simulink model "ProblemSet2"  (R2022a)
settings: Solver=VariableStepAuto  StartTime=0.0  StopTime=10.0  RelTol=1e-3
undefined symbols (not defined in the file): gray
libraries: simulink x4, matrix_library x2, dspindex x2, visiontextngfix x1, visionsources x1
settings Model: Creator=DT  LastModifiedBy=DT

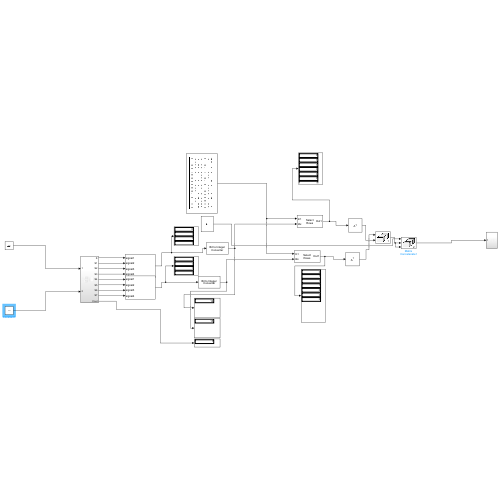
[thumbnail: Simulink's stored preview of the top-level diagram]
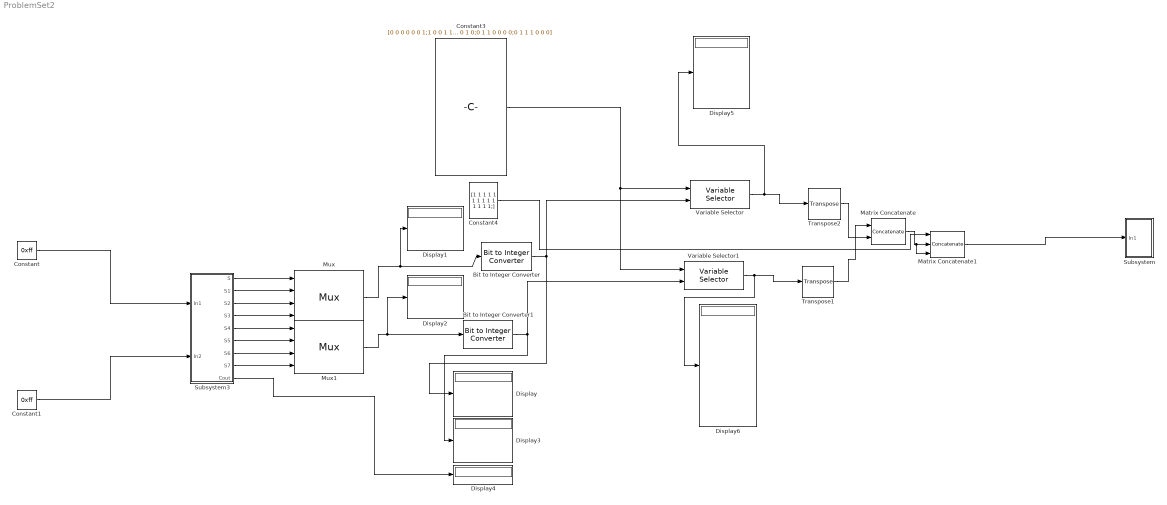
== system ProblemSet2 ==
  Bit to Integer Converter : simulink/Logic and Bit Operations/Bit to Integer Converter  nbits=4  bitOrder=LSB first  signedOutputValues=Unsigned  outDtype=Inherit via internal rule  outDtypeSigned=Inherit via internal rule
      settings: SourceProductBaseCode=SL
  Bit to Integer Converter1 : simulink/Logic and Bit Operations/Bit to Integer Converter  nbits=4  bitOrder=LSB first  signedOutputValues=Unsigned  outDtype=Inherit via internal rule  outDtypeSigned=Inherit via internal rule
      settings: SourceProductBaseCode=SL
  Constant : Constant  Value=0xff
  Constant1 : Constant  Value=0xff
  Constant3 : Constant  Value=[0 0 0 0 0 0 1;1 0 0 1 1 1 1;0 0 1 0 0 1 0;0 0 0 0 1 1 0;1 0 0 1 1 0 0;0 1 0 0 1 0 0 ;0 1 0 0 0 0 0;0 0 0 1 1 1 1;0 0 0 0 0 0 0;0 0 0 0 1 0 0;0 0 0 1 0 0 0;1 1 0 0 0 0 0;0 1 1 0 0 0 1;1 0 0 0 0 1 0;0 1 1 0 0 0 0;0 1 1 1 0 0 0]
  Constant4 : Constant  Value=[1 1 1 1 1 1 1 1 1 1 1 1 1 1;]
  Display{,1..6} (7 alike) : Display
      Display settings: Decimation=8
      Display3 settings: Decimation=8
  Matrix Concatenate : Concatenate  Mode=Multidimensional array
  Matrix Concatenate1 : Concatenate  NumInputs=3  Mode=Multidimensional array  ConcatenateDimension=2
  Mux : Mux
      settings: DisplayOption=signals
  Mux1 : Mux
      settings: DisplayOption=signals
  Subsystem : Subsystem
  Subsystem3 : Subsystem
  Transpose1 : matrix_library/Transpose
      settings: SourceProductBaseCode=SL
  Transpose2 : matrix_library/Transpose
      settings: SourceProductBaseCode=SL
  Variable Selector : dspindex/Variable Selector  NumInputs=1  rowsOrCols=Rows  IdxMode=Variable  Elements=[1 3]  ZerOneIdxMode=Zero-based  errmode=Clip Index  FillMode=on  FillValues=0
  Variable Selector1 : dspindex/Variable Selector  NumInputs=1  rowsOrCols=Rows  IdxMode=Variable  Elements=[1 3]  ZerOneIdxMode=Zero-based  errmode=Clip Index  FillMode=on  FillValues=0
  wires:
  Constant/1 -> Subsystem3/1(In1)
  Constant1/1 -> Subsystem3/2(In2)
  Subsystem3/1(S) -> Mux/1
  Subsystem3/2(S1) -> Mux/2
  Subsystem3/3(S2) -> Mux/3
  Subsystem3/4(S3) -> Mux/4
  Subsystem3/8(S7) -> Mux1/4
  Subsystem3/5(S4) -> Mux1/1
  Subsystem3/6(S5) -> Mux1/2
  Subsystem3/7(S6) -> Mux1/3
  Mux1/1 -> Display2/1, Bit to Integer Converter1/1
  Bit to Integer Converter/1 -> Display/1, Variable Selector/2
  Mux/1 -> Display1/1, Bit to Integer Converter/1
  Bit to Integer Converter1/1 -> Display3/1, Variable Selector1/2
  Subsystem3/9(Cout) -> Display4/1
  Constant3/1 -> Variable Selector1/1, Variable Selector/1
  Variable Selector/1 -> Display5/1, Transpose2/1
  Variable Selector1/1 -> Display6/1, Transpose1/1
  Transpose2/1 -> Matrix Concatenate/2
  Transpose1/1 -> Matrix Concatenate/1
  Matrix Concatenate/1 -> Matrix Concatenate1/3, Matrix Concatenate1/2
  Constant4/1 -> Matrix Concatenate1/1
  Matrix Concatenate1/1 -> Subsystem/1(In1)

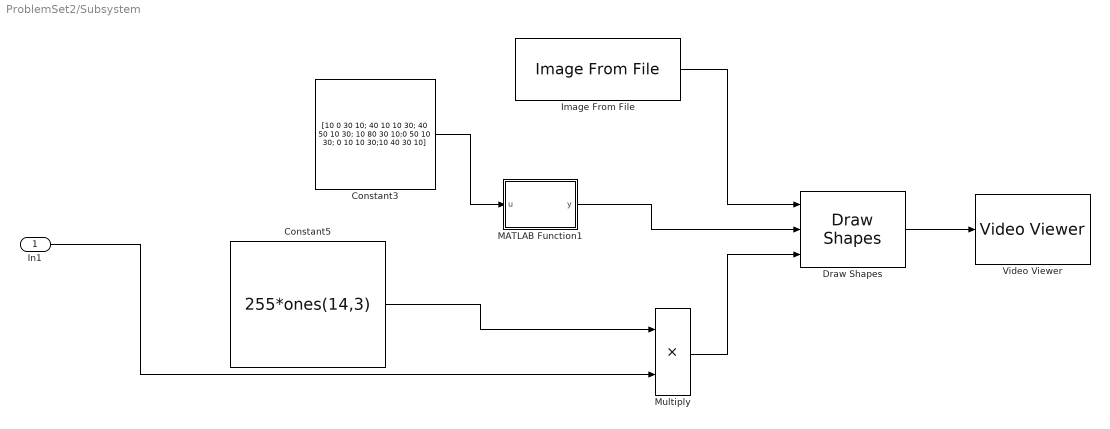
== system ProblemSet2/Subsystem ==
  In1 : Inport
  Constant3 : Constant  Value="[10 0  30 10; 40 10 10 30; 40 50 10 30; 10 80 30 10;0 50 10 30; 0 10 10 30;10 40 30 10]"  VectorParams1D=off
  Constant5 : Constant  Value=255*ones(14,3)
  Draw Shapes : visiontextngfix/Draw Shapes  shape=Rectangles  fill=on  lineWidth=1  fillClrSource=Input port  display=Black  intensity=200  color=[200 255 100]  opacity=0.6  viewport=Entire image  antialiasing=off  inType=Obsolete  imagePorts=One multidimensional signal  roundingMode=Floor  overflowMode=off  memoryMode=Specify word length  memoryWordLength=16  prodOutputMode=Binary point scaling  prodOutputWordLength=32  prodOutputFracLength=14  memoryFracLength=14
  Image From File : visionsources/Image From File  Tag=vipblks_nd  FileName=C:\Users\DT\Downloads\WhiteBackground.png  Ts=inf  imagePorts=One multidimensional signal  OutPortLabels=R|G|B  ImageDataType=double  sdImageDataType=uint(8)  Signed=on  WordLength=16  FractionLengthMode=User-defined  FractionLength=15
  MATLAB Function1 : MATLAB Function  TreatAsAtomicUnit=on
  Multiply : Product
  Video Viewer : VideoViewer  colormapValue=gray(256)  FigPos=[1 814 1536 716]
  wires:
  Constant5/1 -> Multiply/1
  Draw Shapes/1 -> Video Viewer/1
  MATLAB Function1/1(y) -> Draw Shapes/2
  In1/1 -> Multiply/2
  Image From File/1 -> Draw Shapes/1
  Constant3/1 -> MATLAB Function1/1(u)
  Multiply/1 -> Draw Shapes/3

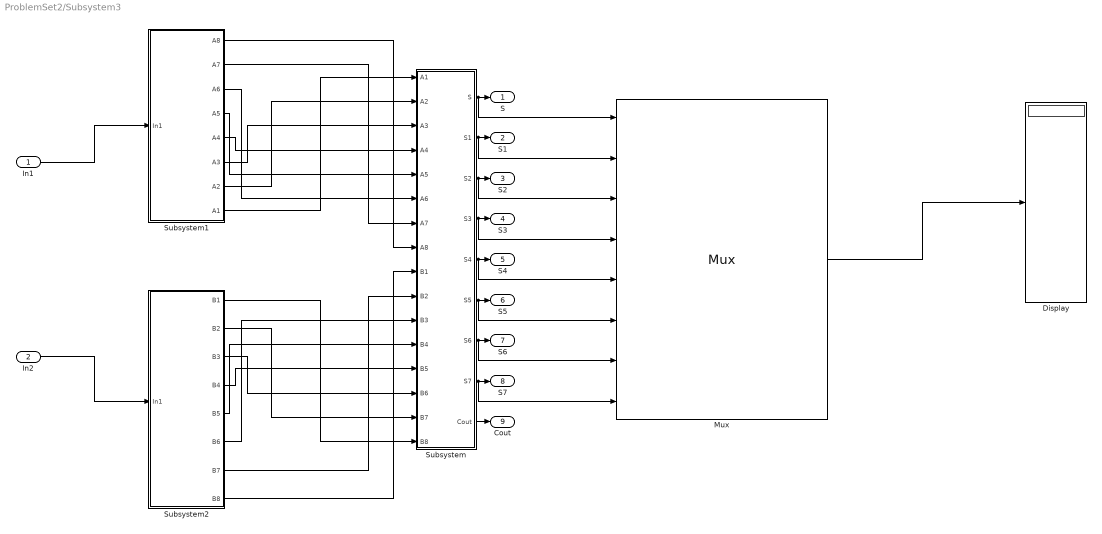
== system ProblemSet2/Subsystem3 ==
  In1 : Inport
  In2 : Inport  Port=2
  Display : Display
  Mux : Mux  Inputs=8
  Subsystem : Subsystem
  Subsystem1 : Subsystem
  Subsystem2 : Subsystem
  S : Outport
  S1 : Outport  Port=2
  S2 : Outport  Port=3
  S3 : Outport  Port=4
  S4 : Outport  Port=5
  S5 : Outport  Port=6
  S6 : Outport  Port=7
  S7 : Outport  Port=8
  Cout : Outport  Port=9
  wires:
  Subsystem/6(S5) -> Mux/6, S5/1
  Subsystem/4(S3) -> Mux/4, S3/1
  In1/1 -> Subsystem1/1(In1)
  In2/1 -> Subsystem2/1(In1)
  Subsystem/5(S4) -> Mux/5, S4/1
  Subsystem/7(S6) -> Mux/7, S6/1
  Subsystem/9(Cout) -> Cout/1
  Subsystem/8(S7) -> Mux/8, S7/1
  Subsystem/2(S1) -> Mux/2, S1/1
  Subsystem/3(S2) -> Mux/3, S2/1
  Subsystem/1(S) -> Mux/1, S/1
  Mux/1 -> Display/1
  Subsystem1/8(A1) -> Subsystem/1(A1)
  Subsystem1/7(A2) -> Subsystem/2(A2)
  Subsystem1/6(A3) -> Subsystem/3(A3)
  Subsystem1/5(A4) -> Subsystem/4(A4)
  Subsystem1/4(A5) -> Subsystem/5(A5)
  Subsystem1/3(A6) -> Subsystem/6(A6)
  Subsystem1/2(A7) -> Subsystem/7(A7)
  Subsystem1/1(A8) -> Subsystem/8(A8)
  Subsystem2/1(B1) -> Subsystem/16(B8)
  Subsystem2/2(B2) -> Subsystem/15(B7)
  Subsystem2/3(B3) -> Subsystem/14(B6)
  Subsystem2/4(B4) -> Subsystem/13(B5)
  Subsystem2/5(B5) -> Subsystem/12(B4)
  Subsystem2/6(B6) -> Subsystem/11(B3)
  Subsystem2/7(B7) -> Subsystem/10(B2)
  Subsystem2/8(B8) -> Subsystem/9(B1)

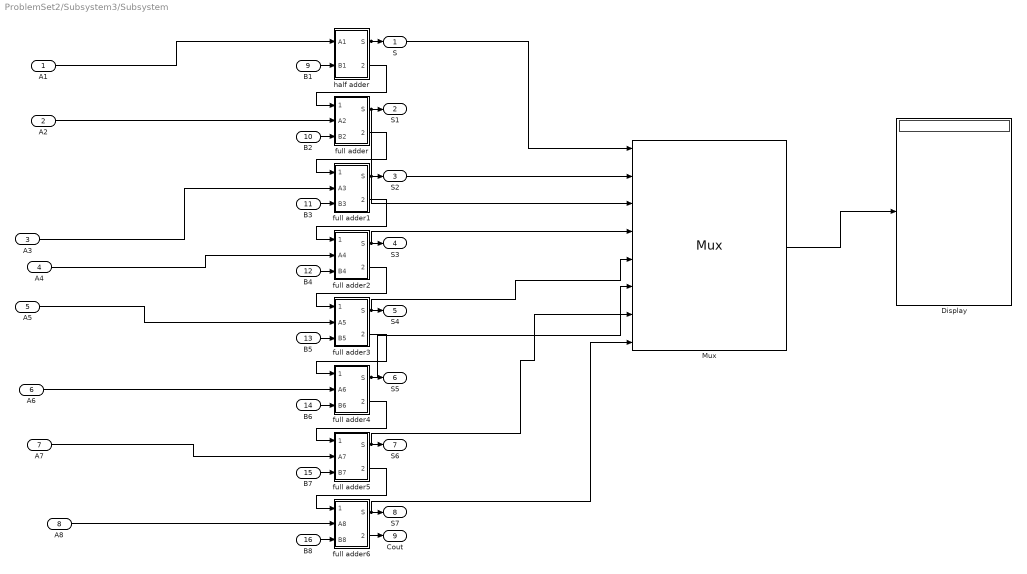
== system ProblemSet2/Subsystem3/Subsystem ==
  A1 : Inport
  A2 : Inport  Port=2
  A3 : Inport  Port=3
  A4 : Inport  Port=4
  A5 : Inport  Port=5
  A6 : Inport  Port=6
  A7 : Inport  Port=7
  A8 : Inport  Port=8
  B1 : Inport  Port=9
  B2 : Inport  Port=10
  B3 : Inport  Port=11
  B4 : Inport  Port=12
  B5 : Inport  Port=13
  B6 : Inport  Port=14
  B7 : Inport  Port=15
  B8 : Inport  Port=16
  Display : Display
  Mux : Mux  Inputs=8
  full adder : Subsystem
  full adder1 : Subsystem
  full adder2 : Subsystem
  full adder3 : Subsystem
  full adder4 : Subsystem
  full adder5 : Subsystem
  full adder6 : Subsystem
  half adder : Subsystem
  S : Outport
  S1 : Outport  Port=2
  S2 : Outport  Port=3
  S3 : Outport  Port=4
  S4 : Outport  Port=5
  S5 : Outport  Port=6
  S6 : Outport  Port=7
  S7 : Outport  Port=8
  Cout : Outport  Port=9
  wires:
  A7/1 -> full adder5/2(A7)
  A8/1 -> full adder6/2(A8)
  full adder6/1(S) -> Mux/8, S7/1
  full adder1/2(Cout) -> full adder2/1(Cin)
  full adder4/2(Cout) -> full adder5/1(Cin)
  half adder/2(Cout) -> full adder/1(Cin)
  A6/1 -> full adder4/2(A6)
  full adder2/2(Cout) -> full adder3/1(Cin)
  full adder5/2(Cout) -> full adder6/1(Cin)
  full adder/2(Cout) -> full adder1/1(Cin)
  full adder2/1(S) -> Mux/4, S3/1
  A3/1 -> full adder1/2(A3)
  full adder3/2(Cout) -> full adder4/1(Cin)
  A2/1 -> full adder/2(A2)
  A1/1 -> half adder/1(A1)
  A4/1 -> full adder2/2(A4)
  full adder/1(S) -> Mux/2, S1/1
  B3/1 -> full adder1/3(B3)
  A5/1 -> full adder3/2(A5)
  B6/1 -> full adder4/3(B6)
  full adder4/1(S) -> Mux/6, S5/1
  B7/1 -> full adder5/3(B7)
  half adder/1(S) -> Mux/1, S/1
  full adder5/1(S) -> Mux/7, S6/1
  full adder6/2(Cout) -> Cout/1
  B1/1 -> half adder/2(B1)
  B8/1 -> full adder6/3(B8)
  B4/1 -> full adder2/3(B4)
  full adder1/1(S) -> Mux/3, S2/1
  full adder3/1(S) -> Mux/5, S4/1
  B2/1 -> full adder/3(B2)
  B5/1 -> full adder3/3(B5)
  Mux/1 -> Display/1

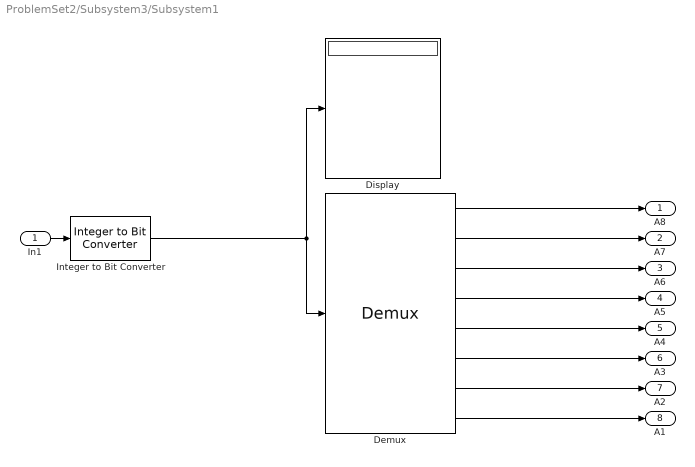
== system ProblemSet2/Subsystem3/Subsystem1 ==
  In1 : Inport
  Demux : Demux  Outputs=8
  Display : Display
  Integer to Bit Converter : simulink/Logic and Bit Operations/Integer to Bit Converter  nbits=8  signedInputValues=Unsigned  bitOrder=MSB first  outDtype=Inherit via internal rule
      settings: SourceProductBaseCode=SL
  A8 : Outport
  A7 : Outport  Port=2
  A6 : Outport  Port=3
  A5 : Outport  Port=4
  A4 : Outport  Port=5
  A3 : Outport  Port=6
  A2 : Outport  Port=7
  A1 : Outport  Port=8
  wires:
  Integer to Bit Converter/1 -> Display/1, Demux/1
  In1/1 -> Integer to Bit Converter/1
  Demux/1 -> A8/1
  Demux/2 -> A7/1
  Demux/3 -> A6/1
  Demux/4 -> A5/1
  Demux/5 -> A4/1
  Demux/6 -> A3/1
  Demux/7 -> A2/1
  Demux/8 -> A1/1

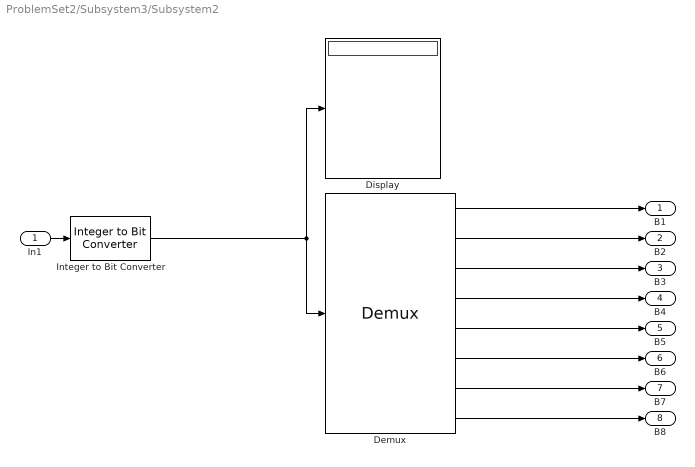
== system ProblemSet2/Subsystem3/Subsystem2 ==
  In1 : Inport
  Demux : Demux  Outputs=8
  Display : Display
  Integer to Bit Converter : simulink/Logic and Bit Operations/Integer to Bit Converter  nbits=8  signedInputValues=Unsigned  bitOrder=MSB first  outDtype=Inherit via internal rule
      settings: SourceProductBaseCode=SL
  B1 : Outport
  B2 : Outport  Port=2
  B3 : Outport  Port=3
  B4 : Outport  Port=4
  B5 : Outport  Port=5
  B6 : Outport  Port=6
  B7 : Outport  Port=7
  B8 : Outport  Port=8
  wires:
  Integer to Bit Converter/1 -> Display/1, Demux/1
  In1/1 -> Integer to Bit Converter/1
  Demux/1 -> B1/1
  Demux/2 -> B2/1
  Demux/3 -> B3/1
  Demux/4 -> B4/1
  Demux/5 -> B5/1
  Demux/6 -> B6/1
  Demux/7 -> B7/1
  Demux/8 -> B8/1

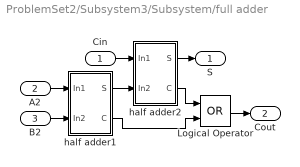
== system ProblemSet2/Subsystem3/Subsystem/full adder ==
  Cin : Inport
  A2 : Inport  Port=2
  B2 : Inport  Port=3
  Logical Operator : Logic  Operator=OR  AllPortsSameDT=off  OutDataTypeStr=boolean
  half adder1 : Subsystem
  half adder2 : Subsystem
  S : Outport
  Cout : Outport  Port=2
  wires:
  half adder1/1(S) -> half adder2/2(In2)
  half adder1/2(C) -> Logical Operator/2
  Logical Operator/1 -> Cout/1
  half adder2/1(S) -> S/1
  half adder2/2(C) -> Logical Operator/1
  Cin/1 -> half adder2/1(In1)
  A2/1 -> half adder1/1(In1)
  B2/1 -> half adder1/2(In2)

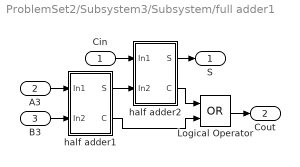
== system ProblemSet2/Subsystem3/Subsystem/full adder1 ==
  Cin : Inport
  A3 : Inport  Port=2
  B3 : Inport  Port=3
  Logical Operator : Logic  Operator=OR  AllPortsSameDT=off  OutDataTypeStr=boolean
  half adder1 : Subsystem
  half adder2 : Subsystem
  S : Outport
  Cout : Outport  Port=2
  wires:
  half adder1/1(S) -> half adder2/2(In2)
  half adder1/2(C) -> Logical Operator/2
  Logical Operator/1 -> Cout/1
  half adder2/1(S) -> S/1
  half adder2/2(C) -> Logical Operator/1
  Cin/1 -> half adder2/1(In1)
  A3/1 -> half adder1/1(In1)
  B3/1 -> half adder1/2(In2)

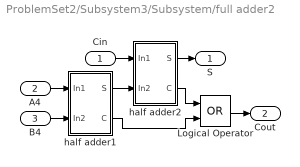
== system ProblemSet2/Subsystem3/Subsystem/full adder2 ==
  Cin : Inport
  A4 : Inport  Port=2
  B4 : Inport  Port=3
  Logical Operator : Logic  Operator=OR  AllPortsSameDT=off  OutDataTypeStr=boolean
  half adder1 : Subsystem
  half adder2 : Subsystem
  S : Outport
  Cout : Outport  Port=2
  wires:
  half adder1/1(S) -> half adder2/2(In2)
  half adder1/2(C) -> Logical Operator/2
  Logical Operator/1 -> Cout/1
  half adder2/1(S) -> S/1
  half adder2/2(C) -> Logical Operator/1
  Cin/1 -> half adder2/1(In1)
  A4/1 -> half adder1/1(In1)
  B4/1 -> half adder1/2(In2)

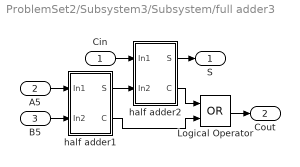
== system ProblemSet2/Subsystem3/Subsystem/full adder3 ==
  Cin : Inport
  A5 : Inport  Port=2
  B5 : Inport  Port=3
  Logical Operator : Logic  Operator=OR  AllPortsSameDT=off  OutDataTypeStr=boolean
  half adder1 : Subsystem
  half adder2 : Subsystem
  S : Outport
  Cout : Outport  Port=2
  wires:
  half adder1/1(S) -> half adder2/2(In2)
  half adder1/2(C) -> Logical Operator/2
  Logical Operator/1 -> Cout/1
  half adder2/1(S) -> S/1
  half adder2/2(C) -> Logical Operator/1
  Cin/1 -> half adder2/1(In1)
  A5/1 -> half adder1/1(In1)
  B5/1 -> half adder1/2(In2)

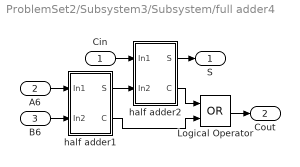
== system ProblemSet2/Subsystem3/Subsystem/full adder4 ==
  Cin : Inport
  A6 : Inport  Port=2
  B6 : Inport  Port=3
  Logical Operator : Logic  Operator=OR  AllPortsSameDT=off  OutDataTypeStr=boolean
  half adder1 : Subsystem
  half adder2 : Subsystem
  S : Outport
  Cout : Outport  Port=2
  wires:
  half adder1/1(S) -> half adder2/2(In2)
  half adder1/2(C) -> Logical Operator/2
  Logical Operator/1 -> Cout/1
  half adder2/1(S) -> S/1
  half adder2/2(C) -> Logical Operator/1
  Cin/1 -> half adder2/1(In1)
  A6/1 -> half adder1/1(In1)
  B6/1 -> half adder1/2(In2)

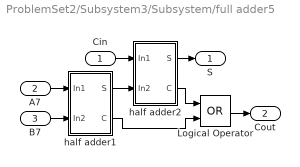
== system ProblemSet2/Subsystem3/Subsystem/full adder5 ==
  Cin : Inport
  A7 : Inport  Port=2
  B7 : Inport  Port=3
  Logical Operator : Logic  Operator=OR  AllPortsSameDT=off  OutDataTypeStr=boolean
  half adder1 : Subsystem
  half adder2 : Subsystem
  S : Outport
  Cout : Outport  Port=2
  wires:
  half adder1/1(S) -> half adder2/2(In2)
  half adder1/2(C) -> Logical Operator/2
  Logical Operator/1 -> Cout/1
  half adder2/1(S) -> S/1
  half adder2/2(C) -> Logical Operator/1
  Cin/1 -> half adder2/1(In1)
  A7/1 -> half adder1/1(In1)
  B7/1 -> half adder1/2(In2)

== system ProblemSet2/Subsystem3/Subsystem/full adder6 ==
  Cin : Inport
  A8 : Inport  Port=2
  B8 : Inport  Port=3
  Logical Operator : Logic  Operator=OR  AllPortsSameDT=off  OutDataTypeStr=boolean
  half adder1 : Subsystem
  half adder2 : Subsystem
  S : Outport
  Cout : Outport  Port=2
  wires:
  half adder1/1(S) -> half adder2/2(In2)
  half adder1/2(C) -> Logical Operator/2
  Logical Operator/1 -> Cout/1
  half adder2/1(S) -> S/1
  half adder2/2(C) -> Logical Operator/1
  Cin/1 -> half adder2/1(In1)
  A8/1 -> half adder1/1(In1)
  B8/1 -> half adder1/2(In2)

== system ProblemSet2/Subsystem3/Subsystem/half adder ==
  A1 : Inport
  B1 : Inport  Port=2
  Logical Operator2 : Logic  Operator=XOR  AllPortsSameDT=off  OutDataTypeStr=boolean
  Logical Operator3 : Logic  AllPortsSameDT=off  OutDataTypeStr=boolean
  S : Outport
  Cout : Outport  Port=2
  wires:
  B1/1 -> Logical Operator2/2, Logical Operator3/2
  Logical Operator2/1 -> S/1
  A1/1 -> Logical Operator3/1, Logical Operator2/1
  Logical Operator3/1 -> Cout/1

== system ProblemSet2/Subsystem3/Subsystem/full adder/half adder1 ==
  In1 : Inport
  In2 : Inport  Port=2
  Logical Operator2 : Logic  Operator=XOR  AllPortsSameDT=off  OutDataTypeStr=boolean
  Logical Operator3 : Logic  AllPortsSameDT=off  OutDataTypeStr=boolean
  S : Outport
  C : Outport  Port=2
  wires:
  In2/1 -> Logical Operator2/2, Logical Operator3/2
  Logical Operator2/1 -> S/1
  In1/1 -> Logical Operator3/1, Logical Operator2/1
  Logical Operator3/1 -> C/1

== system ProblemSet2/Subsystem3/Subsystem/full adder/half adder2 ==
  In1 : Inport
  In2 : Inport  Port=2
  Logical Operator2 : Logic  Operator=XOR  AllPortsSameDT=off  OutDataTypeStr=boolean
  Logical Operator3 : Logic  AllPortsSameDT=off  OutDataTypeStr=boolean
  S : Outport
  C : Outport  Port=2
  wires:
  In2/1 -> Logical Operator2/2, Logical Operator3/2
  Logical Operator2/1 -> S/1
  In1/1 -> Logical Operator3/1, Logical Operator2/1
  Logical Operator3/1 -> C/1

== system ProblemSet2/Subsystem3/Subsystem/full adder1/half adder1 ==
  In1 : Inport
  In2 : Inport  Port=2
  Logical Operator2 : Logic  Operator=XOR  AllPortsSameDT=off  OutDataTypeStr=boolean
  Logical Operator3 : Logic  AllPortsSameDT=off  OutDataTypeStr=boolean
  S : Outport
  C : Outport  Port=2
  wires:
  In2/1 -> Logical Operator2/2, Logical Operator3/2
  Logical Operator2/1 -> S/1
  In1/1 -> Logical Operator3/1, Logical Operator2/1
  Logical Operator3/1 -> C/1

== system ProblemSet2/Subsystem3/Subsystem/full adder1/half adder2 ==
  In1 : Inport
  In2 : Inport  Port=2
  Logical Operator2 : Logic  Operator=XOR  AllPortsSameDT=off  OutDataTypeStr=boolean
  Logical Operator3 : Logic  AllPortsSameDT=off  OutDataTypeStr=boolean
  S : Outport
  C : Outport  Port=2
  wires:
  In2/1 -> Logical Operator2/2, Logical Operator3/2
  Logical Operator2/1 -> S/1
  In1/1 -> Logical Operator3/1, Logical Operator2/1
  Logical Operator3/1 -> C/1

== system ProblemSet2/Subsystem3/Subsystem/full adder2/half adder1 ==
  In1 : Inport
  In2 : Inport  Port=2
  Logical Operator2 : Logic  Operator=XOR  AllPortsSameDT=off  OutDataTypeStr=boolean
  Logical Operator3 : Logic  AllPortsSameDT=off  OutDataTypeStr=boolean
  S : Outport
  C : Outport  Port=2
  wires:
  In2/1 -> Logical Operator2/2, Logical Operator3/2
  Logical Operator2/1 -> S/1
  In1/1 -> Logical Operator3/1, Logical Operator2/1
  Logical Operator3/1 -> C/1

== system ProblemSet2/Subsystem3/Subsystem/full adder2/half adder2 ==
  In1 : Inport
  In2 : Inport  Port=2
  Logical Operator2 : Logic  Operator=XOR  AllPortsSameDT=off  OutDataTypeStr=boolean
  Logical Operator3 : Logic  AllPortsSameDT=off  OutDataTypeStr=boolean
  S : Outport
  C : Outport  Port=2
  wires:
  In2/1 -> Logical Operator2/2, Logical Operator3/2
  Logical Operator2/1 -> S/1
  In1/1 -> Logical Operator3/1, Logical Operator2/1
  Logical Operator3/1 -> C/1

== system ProblemSet2/Subsystem3/Subsystem/full adder3/half adder1 ==
  In1 : Inport
  In2 : Inport  Port=2
  Logical Operator2 : Logic  Operator=XOR  AllPortsSameDT=off  OutDataTypeStr=boolean
  Logical Operator3 : Logic  AllPortsSameDT=off  OutDataTypeStr=boolean
  S : Outport
  C : Outport  Port=2
  wires:
  In2/1 -> Logical Operator2/2, Logical Operator3/2
  Logical Operator2/1 -> S/1
  In1/1 -> Logical Operator3/1, Logical Operator2/1
  Logical Operator3/1 -> C/1

== system ProblemSet2/Subsystem3/Subsystem/full adder3/half adder2 ==
  In1 : Inport
  In2 : Inport  Port=2
  Logical Operator2 : Logic  Operator=XOR  AllPortsSameDT=off  OutDataTypeStr=boolean
  Logical Operator3 : Logic  AllPortsSameDT=off  OutDataTypeStr=boolean
  S : Outport
  C : Outport  Port=2
  wires:
  In2/1 -> Logical Operator2/2, Logical Operator3/2
  Logical Operator2/1 -> S/1
  In1/1 -> Logical Operator3/1, Logical Operator2/1
  Logical Operator3/1 -> C/1

== system ProblemSet2/Subsystem3/Subsystem/full adder4/half adder1 ==
  In1 : Inport
  In2 : Inport  Port=2
  Logical Operator2 : Logic  Operator=XOR  AllPortsSameDT=off  OutDataTypeStr=boolean
  Logical Operator3 : Logic  AllPortsSameDT=off  OutDataTypeStr=boolean
  S : Outport
  C : Outport  Port=2
  wires:
  In2/1 -> Logical Operator2/2, Logical Operator3/2
  Logical Operator2/1 -> S/1
  In1/1 -> Logical Operator3/1, Logical Operator2/1
  Logical Operator3/1 -> C/1

== system ProblemSet2/Subsystem3/Subsystem/full adder4/half adder2 ==
  In1 : Inport
  In2 : Inport  Port=2
  Logical Operator2 : Logic  Operator=XOR  AllPortsSameDT=off  OutDataTypeStr=boolean
  Logical Operator3 : Logic  AllPortsSameDT=off  OutDataTypeStr=boolean
  S : Outport
  C : Outport  Port=2
  wires:
  In2/1 -> Logical Operator2/2, Logical Operator3/2
  Logical Operator2/1 -> S/1
  In1/1 -> Logical Operator3/1, Logical Operator2/1
  Logical Operator3/1 -> C/1

== system ProblemSet2/Subsystem3/Subsystem/full adder5/half adder1 ==
  In1 : Inport
  In2 : Inport  Port=2
  Logical Operator2 : Logic  Operator=XOR  AllPortsSameDT=off  OutDataTypeStr=boolean
  Logical Operator3 : Logic  AllPortsSameDT=off  OutDataTypeStr=boolean
  S : Outport
  C : Outport  Port=2
  wires:
  In2/1 -> Logical Operator2/2, Logical Operator3/2
  Logical Operator2/1 -> S/1
  In1/1 -> Logical Operator3/1, Logical Operator2/1
  Logical Operator3/1 -> C/1

== system ProblemSet2/Subsystem3/Subsystem/full adder5/half adder2 ==
  In1 : Inport
  In2 : Inport  Port=2
  Logical Operator2 : Logic  Operator=XOR  AllPortsSameDT=off  OutDataTypeStr=boolean
  Logical Operator3 : Logic  AllPortsSameDT=off  OutDataTypeStr=boolean
  S : Outport
  C : Outport  Port=2
  wires:
  In2/1 -> Logical Operator2/2, Logical Operator3/2
  Logical Operator2/1 -> S/1
  In1/1 -> Logical Operator3/1, Logical Operator2/1
  Logical Operator3/1 -> C/1

== system ProblemSet2/Subsystem3/Subsystem/full adder6/half adder1 ==
  In1 : Inport
  In2 : Inport  Port=2
  Logical Operator2 : Logic  Operator=XOR  AllPortsSameDT=off  OutDataTypeStr=boolean
  Logical Operator3 : Logic  AllPortsSameDT=off  OutDataTypeStr=boolean
  S : Outport
  C : Outport  Port=2
  wires:
  In2/1 -> Logical Operator2/2, Logical Operator3/2
  Logical Operator2/1 -> S/1
  In1/1 -> Logical Operator3/1, Logical Operator2/1
  Logical Operator3/1 -> C/1

== system ProblemSet2/Subsystem3/Subsystem/full adder6/half adder2 ==
  In1 : Inport
  In2 : Inport  Port=2
  Logical Operator2 : Logic  Operator=XOR  AllPortsSameDT=off  OutDataTypeStr=boolean
  Logical Operator3 : Logic  AllPortsSameDT=off  OutDataTypeStr=boolean
  S : Outport
  C : Outport  Port=2
  wires:
  In2/1 -> Logical Operator2/2, Logical Operator3/2
  Logical Operator2/1 -> S/1
  In1/1 -> Logical Operator3/1, Logical Operator2/1
  Logical Operator3/1 -> C/1

== matlab function ProblemSet2/Subsystem/MATLAB Function1 ==
  data: u input; y output
function y = fcn(u)
v = repmat([60 0 0 0],7,1)
v = u+v;
y = [u;v];
